simulink model "CT_CPC2_nivel"  (Simulink 8.1)
settings: Solver=ode45  StartTime=0.0  StopTime=60  FixedStep=Tm  RelTol=1e-3
InitFcn:
  | Tm = 0.01;
settings Model: Creator=Equipo-Servo  LastModifiedBy=Equipo-Servo  ExtModeTrigDuration=100000
settings DataIOCC: SignalLoggingSaveFormat=Dataset
settings OptimizationCC: ExpressionDepthLimit=128
settings DebuggingCC: FcnCallInpInsideContextMsg=EnableAllAsError
settings HardwareCC: ProdIntDivRoundTo=Zero  ProdEndianess=LittleEndian  ProdHWDeviceType=Generic->32-bit x86 compatible
settings RTWCC: SystemTargetFile=rtwin.tlc  TemplateMakefile=rtwin.tmf  Description=Real-Time Windows Target  ProcessScript=rtwin_make_rtw_hook  RTWCompilerOptimization=On
settings CodeAppCC: MaxIdLength=95
settings RTWinTargetCC: TargetLibSuffix=_rtwin.lib  TargetPreCompLibLocation=C:\Program Files\MATLAB\R2013a\toolbox\rtw\targets\rtwin\lib\win32  CodeReplacementLibrary=ANSI_C  RTWinDir=C:/PROGRA~1/MATLAB/R2013a/toolbox/rtw/targets/rtwin  TargetArch=win32

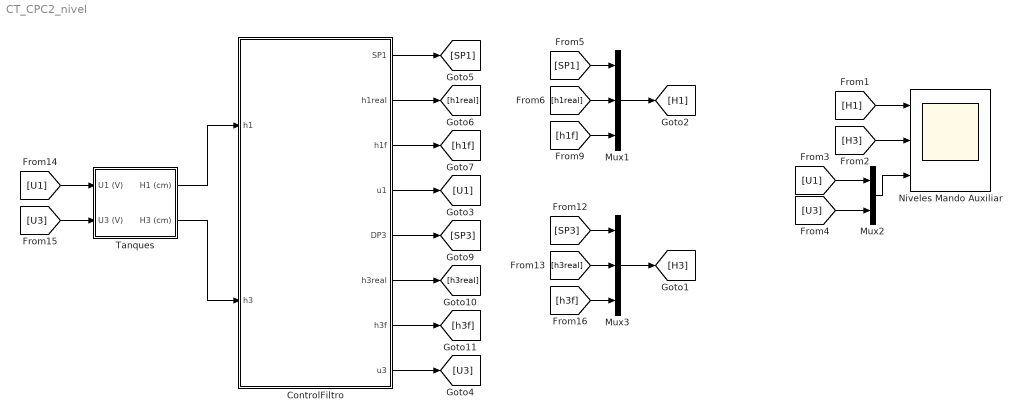
== system CT_CPC2_nivel ==
  ControlFiltro : Subsystem
  Mux1 : Mux  Inputs=3
  Mux2 : Mux  Inputs=2
  Mux3 : Mux  Inputs=3
  Niveles Mando Auxiliar : Scope  NumInputPorts=3
      settings: TimeRange=60  YMin=8.5~8~-5  YMax=17~16.5~55
  Tanques : Subsystem
  wires:
  [U1] -> Tanques/1(U1 (V))
  [U3] -> Tanques/2(U3 (V))
  Mux1/1 -> [H1]
  ControlFiltro/4(u1) -> [U1]
  ControlFiltro/8(u3) -> [U3]
  ControlFiltro/1(SP1) -> [SP1]
  ControlFiltro/2(h1real) -> [h1real]
  ControlFiltro/3(h1f) -> [h1f]
  [h1real] -> Mux1/2
  [SP1] -> Mux1/1
  [h1f] -> Mux1/3
  Mux3/1 -> [H3]
  [h3real] -> Mux3/2
  [SP3] -> Mux3/1
  [h3f] -> Mux3/3
  ControlFiltro/5(DP3) -> [SP3]
  ControlFiltro/6(h3real) -> [h3real]
  ControlFiltro/7(h3f) -> [h3f]
  Tanques/1(H1 (cm)) -> ControlFiltro/1(h1)
  Tanques/2(H3 (cm)) -> ControlFiltro/2(h3)
  [H1] -> Niveles Mando Auxiliar/1
  [H3] -> Niveles Mando Auxiliar/2
  [U1] -> Mux2/1
  [U3] -> Mux2/2
  Mux2/1 -> Niveles Mando Auxiliar/3

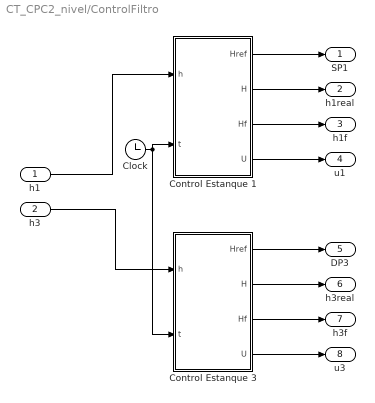
== system CT_CPC2_nivel/ControlFiltro ==
  h1 : Inport
  h3 : Inport  Port=2
  Clock : Clock
  Control Estanque 1 : MATLAB Function  TreatAsAtomicUnit=on
  Control Estanque 3 : MATLAB Function  TreatAsAtomicUnit=on
  SP1 : Outport
  h1real : Outport  Port=2
  h1f : Outport  Port=3
  u1 : Outport  Port=4
  DP3 : Outport  Port=5
  h3real : Outport  Port=6
  h3f : Outport  Port=7
  u3 : Outport  Port=8
  wires:
  Clock/1 -> Control Estanque 3/2(t), Control Estanque 1/2(t)
  Control Estanque 3/4(U) -> u3/1
  Control Estanque 3/3(Hf) -> h3f/1
  Control Estanque 3/2(H) -> h3real/1
  Control Estanque 3/1(Href) -> DP3/1
  Control Estanque 1/4(U) -> u1/1
  Control Estanque 1/3(Hf) -> h1f/1
  Control Estanque 1/2(H) -> h1real/1
  Control Estanque 1/1(Href) -> SP1/1
  h1/1 -> Control Estanque 1/1(h)
  h3/1 -> Control Estanque 3/1(h)

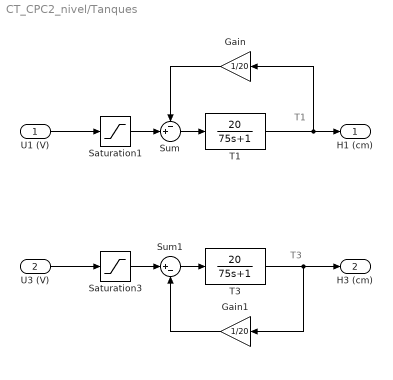
== system CT_CPC2_nivel/Tanques ==
  note: T3
  note: T1
  U1 (V) : Inport
  U3 (V) : Inport  Port=2
  Gain : Gain  Gain=1/20
  Gain1 : Gain  Gain=1/20
  Saturation1 : Saturate  UpperLimit=5  LowerLimit=0
  Saturation3 : Saturate  UpperLimit=5  LowerLimit=0
  Sum : Sum  Inputs=-+|
  Sum1 : Sum  Inputs=|+-
  T1 : TransferFcn  Numerator=[20]  Denominator=[75 1]
  T3 : TransferFcn  Numerator=[20]  Denominator=[75 1]
  H1 (cm) : Outport
  H3 (cm) : Outport  Port=2
  wires:
  T1/1 -> Gain/1, H1 (cm)/1
  U1 (V)/1 -> Saturation1/1
  U3 (V)/1 -> Saturation3/1
  T3/1 -> Gain1/1, H3 (cm)/1
  Saturation1/1 -> Sum/2
  Sum/1 -> T1/1
  Gain/1 -> Sum/1
  Saturation3/1 -> Sum1/1
  Sum1/1 -> T3/1
  Gain1/1 -> Sum1/2

== matlab function ControlFiltro/Control Estanque 3 ==
  data: h input double; Href output double; H output double; Hf output double; U output double; t input double
function [Href,H,Hf,U] = fcn(h,t)

Tm = 0.5;
alpha = exp(-1*Tm);
persistent hf
if isempty(hf)
    hf = 0;
end

%% filtro de primer orden
hf = alpha*hf + (1 - alpha)*h;

%% Controlador PID
kc = 5;
Href = 10 + 5*(t>=30);
ek = Href - hf;
u = kc*ek;

%% salidas
H = h;
Hf = hf;
U = u;

== matlab function ControlFiltro/Control Estanque 1 ==
  data: h input double; Href output double; H output double; Hf output double; U output double; t input double
function [Href,H,Hf,U] = fcn(h,t)

Tm = 0.5;
alpha = exp(-1*Tm);
persistent hf
if isempty(hf)
    hf = 0;
end

%% filtro de primer orden
hf = alpha*hf + (1 - alpha)*h;

%% Controlador PID
kc = 10;
Href = 10 + 5*(t>=30);
ek = Href - hf;
u = kc*ek;

%% salidas
H = h;
Hf = hf;
U = u;
